simulink library "Electric_Drive_Tabled_Consumption"  (R2018b)
settings: Solver=VariableStepAuto  StartTime=0.0  StopTime=10.0  RelTol=1e-3
undefined symbols (not defined in the file): OM_PEl_M_Map, PEl_MotVector
(part 1 of 2)
settings Model: Creator=ga69qig  LastModifiedBy=ga69qig
settings SFSimCC: SimUseLocalCustomCode=off
settings RTWCC: RTWUseLocalCustomCode=off

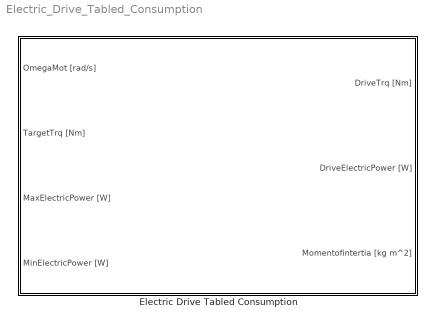
== system Electric_Drive_Tabled_Consumption ==
  Electric Drive Tabled Consumption : Subsystem  mask(SB){inertia=0.03, mass=1, OM_M_Pel_Map=[0 84.6925537915840 106.777901162710 132.451481077187 158.717445659769 189.583562564064 219.947567848300 253.359271731562 287.719734913549 325.267898465954 364.560585120281 403.200274983864 447.563591693892 492.828790386663 540.691726349864 590.166785808662 636.561358483905 684.766906055931 734.137596997731 789.985532553104 857.853179816674 908.827398035181 961.684563108046 1019.52904110769 1081.52112973929 1143.57712046773 1200.78427519799 1267.27434692366 1330.96763225908 1399.91145341150 1460.96283186014 1522.13532912128 1591.13337312260 1654.62568484686 1718.49067047593 1783.14030989899 1852.47991946389 1921.56456923299 1990.91312442103 2061.30678608583 2131.34426123832 2203.05270027821 2289.55226312012 2376.68282420177 2454.52733777355 2530.75949498243 2607.34099640618 2684.42711031811 2763.34508226637 2845.97385304829 2963.00280011347 3052.53326845787 3134.40614789669 3225.26823505504 3314.19457665049 3406.50541394017 3500.20227762135 3591.35102796290 3685.03225906601 3782.98250894227 3881.87095410315 3980.79391338854 4076.30627526000 4181.94930220964 4286.97881720375 4389.92406519024 4497.41842284860 4603.47594352982 4710.85061726193 4818.54315585332 4930.22331092001 5041.15761416958 5166.37122862945 5276.81725954101 5387.76544736434 5521.32616802780 5637.26001511646 5761.43879713315 5886.21150930422 6012.17873781274 6142.71364240950 6280.27669163038 5676.19543942961 5258.13958693589 5295.58110214479 5435.21609088646 5171.11785981694 5274.97483494523 5470.31098908416 5158.84365253269 5768.15695867421 5696.91368959506 6048.96408164810 6479.69942526134 6479.69942526134 6479.69942526134 6479.69942526134 6479.69942526134 6479.69942526134 6479.69942526134;0 84.6925537915840 106.777901162710 132.451481077187 158.717445659769 189.583562564064 219.947567848300 253.359271731562 287.719734913549 325.267898465954 364.560585120281 403.200274983864 447.563591693892 492.828790386663 540.691726349864 590.166785808662 636.561358483905 684.766906055931 734.137596997731 789.985532553104 857.853179816674 908.827398035181 961.684563108046 1019.52904110769 1081.52112973929 1143.57712046773 1200.78427519799 1267.27434692366 1330.96763225908 1399.91145341150 1460.96283186014 1522.13532912128 1591.13337312260 1654.62568484686 1718.49067047593 1783.14030989899 1852.47991946389 1921.56456923299 1990.91312442103 2061.30678608583 2131.34426123832 2203.05270027821 2289.55226312012 2376.68282420177 2454.52733777355 2530.75949498243 2607.34099640618 2684.42711031811 2763.34508226637 2845.97385304829 2963.00280011347 3052.53326845787 3134.40614789669 3225.26823505504 3314.19457665049 3406.50541394017 3500.20227762135 3591.35102796290 3685.03225906601 3782.98250894227 3881.87095410315 3980.79391338854 4076.30627526000 4181.94930220964 4286.97881720375 4389.92406519024 4497.41842284860 4603.47594352982 4710.85061726193 4818.54315585332 4930.22331092001 5041.15761416958 5166.37122862945 5276.81725954101 5387.76544736434 5521.32616802780 5637.26001511646 5761.43879713315 5886.21150930422 6012.17873781274 6142.71364240950 6280.27669163038 5676.19543942961 5258.13958693589 5295.58110214479 5435.21609088646 5171.11785981694 5274.97483494523 5470.31098908416 5158.84365253269 5768.15695867421 5696.91368959506 6048.96408164810 6479.69942526134 6479.69942526134 6479.69942526134 6479.69942526134 6479.69942526134 6479.69942526134 6479.69942526134;0 84.6925537915840 106.777901162710 132.451481077187 158.717445659769 189.583562564064 219.947567848300 253.359271731562 287.719734913549 325.267898465954 364.560585120281 403.200274983864 447.563591693892 492.828790386663 540.691726349864 590.166785808662 636.561358483905 684.766906055931 734.137596997731 789.985532553104 857.853179816674 908.827398035181 961.684563108046 1019.52904110769 1081.52112973929 1143.57712046773 1200.78427519799 1267.27434692366 1330.96763225908 1399.91145341150 1460.96283186014 1522.13532912128 1591.13337312260 1654.62568484686 1718.49067047593 1783.14030989899 1852.47991946389 ...(+366716 chars)], M_MotVector=[0 1.36363636363636 2.72727272727273 4.09090909090909 5.45454545454545 6.81818181818182 8.18181818181818 9.54545454545455 10.9090909090909 12.2727272727273 13.6363636363636 15.0000000000000 16.3636363636364 17.7272727272727 19.0909090909091 20.4545454545455 21.8181818181818 23.1818181818182 24.5454545454545 25.9090909090909 27.2727272727273 28.6363636363636 30.0000000000000 31.3636363636364 32.7272727272727 34.0909090909091 35.4545454545455 36.8181818181818 38.1818181818182 39.5454545454545 40.9090909090909 42.2727272727273 43.6363636363636 45 46.3636363636364 47.7272727272727 49.0909090909091 50.4545454545455 51.8181818181818 53.1818181818182 54.5454545454545 55.9090909090909 57.2727272727273 58.6363636363636 60.0000000000000 61.3636363636364 62.7272727272727 64.0909090909091 65.4545454545455 66.8181818181818 68.1818181818182 69.5454545454546 70.9090909090909 72.2727272727273 73.6363636363636 75 76.3636363636364 77.7272727272727 79.0909090909091 80.4545454545455 81.8181818181818 83.1818181818182 84.5454545454546 85.9090909090909 87.2727272727273 88.6363636363636 90 91.3636363636364 92.7272727272727 94.0909090909091 95.4545454545455 96.8181818181818 98.1818181818182 99.5454545454546 100.909090909091 102.272727272727 103.636363636364 105 106.363636363636 107.727272727273 109.090909090909 110.454545454545 111.818181818182 113.181818181818 114.545454545455 115.909090909091 117.272727272727 118.636363636364 120 121.363636363636 122.727272727273 124.090909090909 125.454545454545 126.818181818182 128.181818181818 129.545454545455 130.909090909091 132.272727272727 133.636363636364 135], OM_MotVector=[0 3.13202920563366 6.26405841126732 9.39608761690098 12.5281168225346 15.6601460281683 18.7921752338020 21.9242044394356 25.0562336450693 28.1882628507029 31.3202920563366 34.4523212619703 37.5843504676039 40.7163796732376 43.8484088788712 46.9804380845049 50.1124672901386 53.2444964957722 56.3765257014059 59.5085549070395 62.6405841126732 65.7726133183069 68.9046425239405 72.0366717295742 75.1687009352078 78.3007301408415 81.4327593464752 84.5647885521088 87.6968177577425 90.8288469633761 93.9608761690098 97.0929053746435 100.224934580277 103.356963785911 106.488992991544 109.621022197178 112.753051402812 115.885080608445 119.017109814079 122.149139019713 125.281168225346 128.413197430980 131.545226636614 134.677255842247 137.809285047881 140.941314253515 144.073343459148 147.205372664782 150.337401870416 153.469431076049 156.601460281683 159.733489487317 162.865518692950 165.997547898584 169.129577104218 172.261606309851 175.393635515485 178.525664721119 181.657693926752 184.789723132386 187.921752338020 191.053781543653 194.185810749287 197.317839954921 200.449869160554 203.581898366188 206.713927571822 209.845956777455 212.977985983089 216.110015188723 219.242044394356 222.374073599990 225.506102805624 228.638132011257 231.770161216891 234.902190422524 238.034219628158 241.166248833792 244.298278039425 247.430307245059 250.562336450693 253.694365656326 256.826394861960 259.958424067594 263.090453273227 266.222482478861 269.354511684495 272.486540890128 275.618570095762 278.750599301396 281.882628507029 285.014657712663 288.146686918297 291.278716123930 294.410745329564 297.542774535198 300.674803740831 303.806832946465 306.938862152099 310.070891357732 313.202920563366 316.334949769000 319.466978974633 322.599008180267 325.731037385901 328.863066591534 331.995095797168 335.127125002802 338.259154208435 341.391183414069 344.523212619703 347.655241825336 350.787271030970 353.919300236604 357.051329442237 360.183358647871 363.315387853505 366.447417059138 369.579446264772 372.711475470406 375.843504676039 378.975533881673 382.107563087307 385.239592292940 388.371621498574 391.503650704208 394.635679909841 397.767709115475 400.899738321108 404.031767526742 407.163796732376 410.295825938009 413.427855143643 416.559884349277 419.691913554910 422.823942760544 425.955971966178 429.088001171811 432.220030377445 435.352059583079 438.484088788712 441.616117994346 444.748147199980 447.880176405613 451.012205611247 454.144234816881 457.276264022514 460.408293228148 463.540322433782 466.672351639415 469.804380845049 472.936410050683 476.068439256316 479.200468461950 482.332497667584 485.464526873217 488.596556078851 491.728585284485 494.860614490118 497.992643695752 501.124672901386 504.256702107019 507.388731312653 510.520760518287 513.652789723920 516.784818929554 519.916848135188 523.048877340821 526.180906546455 529.312935752089 532.444964957722 535.576994163356 538.709023368990 541.841052574623 544.973081780257 548.105110985890 551.237140191524 554.369169397158 557.501198602791 560.633227808425 563.765257014059 566.897286219692 570.029315425326 573.161344630960 576.293373836593 579.425403042227 582.557432247861 585.689461453494 588.821490659128 591.953519864762 595.085549070395 598.217578276029 601.349607481663 604.481636687296 607.613665892930 610.745695098564 613.877724304197 617.009753509831 620.141782715465 623.273811921098 626.405841126732 629.537870332366 632.669899537999 635.801928743633 638.933957949267 642.065987154900 645.198016360534 648.330045566168 651.462074771801 654.594103977435 657.726133183069 660.858162388702 663.990191594336 667.122220799970 670.254250005603 673.386279211237 676.518308416871 679.650337622504 682.782366828138 685.914396033772], M_Full_Load=[128 128 128 127 127 126 126 126 126 124 119 114 109 103 100 94 89 85 79 75 70 68 67 65 63 62 60 58 59 60 62 63 63 62 61 60 58 57 55 53 51 50 48 46 45 43 42 40 39 38 36 35 34 32 31 30 29 28 26 25 24], OM_Full_Load=[0 11.4144533080429 22.8289066160858 34.2433599241288 45.6578132321717 57.1769862953342 68.5914396033771 80.0058929114201 91.4203462194630 102.834799527506 114.249252835549 125.663706143592 137.078159451635 148.492612759678 160.011785822840 171.426239130883 182.840692438926 194.255145746969 205.669599055012 217.084052363055 228.498505671098 239.912958979141 251.327412287183 262.846585350346 274.261038658389 285.675491966432 297.089945274475 308.504398582518 319.918851890561 331.333305198604 342.747758506646 354.162211814689 365.681384877852 377.095838185895 388.510291493938 399.924744801981 411.339198110024 422.753651418066 434.168104726109 445.582558034152 456.997011342195 468.516184405358 479.930637713401 491.345091021444 502.759544329487 514.173997637529 525.588450945572 537.002904253615 548.417357561658 559.831810869701 571.350983932864 582.765437240907 594.179890548950 605.594343856992 617.008797165035 628.423250473078 639.837703781121 651.252157089164 662.666610397207 674.185783460370 685.600236768413], M_Min_Load=[0 0 0 0 0 0 0 0 0 0 0 0 0 0 0 0 0 0 0 0 0 0 0 0 0 0 0 0 0 0 0 0 0 0 0 0 0 0 0 0 0 0 0 0 0 0 0 0 0 0 0 0 0 0 0 0 0 0 0 0 0], OM_Min_Load=[0 11.4144533080429 22.8289066160858 34.2433599241288 45.6578132321717 57.1769862953342 68.5914396033771 80.0058929114201 91.4203462194630 102.834799527506 114.249252835549 125.663706143592 137.078159451635 148.492612759678 160.011785822840 171.426239130883 182.840692438926 194.255145746969 205.669599055012 217.084052363055 228.498505671098 239.912958979141 251.327412287183 262.846585350346 274.261038658389 285.675491966432 297.089945274475 308.504398582518 319.918851890561 331.333305198604 342.747758506646 354.162211814689 365.681384877852 377.095838185895 388.510291493938 399.924744801981 411.339198110024 422.753651418066 434.168104726109 445.582558034152 456.997011342195 468.516184405358 479.930637713401 491.345091021444 502.759544329487 514.173997637529 525.588450945572 537.002904253615 548.417357561658 559.831810869701 571.350983932864 582.765437240907 594.179890548950 605.594343856992 617.008797165035 628.423250473078 639.837703781121 651.252157089164 662.666610397207 674.185783460370 685.600236768413], LocalSampleTime=-1}
      mask prompts: inertia "Moment of Inertia E-Motor [kg*m^2]"; mass "Mass E-Motor [kg"; OM_M_Pel_Map "Tabled Electric Power [NxM]"; M_MotVector "Reference Torque Vector [1xM]"; OM_MotVector "Reference Omega Vector [1xN]"; M_Full_Load "Torque Vector for Full Load Line [1xL]"; OM_Full_Load "Reference Omega Vector for Full Load Line [1xL]"; M_Min_Load "Torque Vector for Min Load Line [1xK]"; OM_Min_Load "Reference Omega Vector for Min Load Line [1xK]"; LocalSampleTime "Local System Sample-Time [s]"
      mask help:
      | <Author> Benedikt Danquah based on Lorenz Horlbeck [1] and Philip Wacker [2]</Author>
      | <Date> 01/2019 </Date>
      |
      | <Description>
      | Calculates the target drive torque. The avaiable max./min. electric power of the battery limits the electric system. The mechanical system is limited by the max./min. torque curve. Due to the limits the final drive torque and the drive electric power (via 2D-Lookup table) is calculated. The moment of inertia is given as a constant signal.
      | </Description>
      mask init:
      | GlobalSampleTime = CalcGlobalSampleTime(LocalSampleTime);
      | 
      | [OM_PEl_M_Map,OM_MotVector, PEl_MotVector]= init_Electric_Drive_Tabled_Consumption (OM_M_Pel_Map,M_MotVector,OM_MotVector,M_Full_Load,OM_Full_Load,M_Min_Load,OM_Min_Load);
      | 
      | %figure
      | %hold on
      | %surfc(OM_MotVector,M_MotVector,OM_M_Pel_Map')
      | %for i=1:1000
      |  %   plot3(OM_Full_Load,M_Full_Load,ones(1,61)*i*30,'color','red', 'linewidth',6)
      | %end
      | %hold off
      | 
      | 
      | %figure
      | %surfc(OM_MotVector,PEl_Vector,OM_PEl_M_Map')
      mask Help:
      | <Parameters>
      | Moment of Inertia E-Motor [kg*m^2]
      | Mass E-Motor [kg]
      | Tabled Electric Power [NxM]
      | Reference Torque Vector [1xM]
      | Reference Omega Vector [1xN]
      | Torque Vector for Full Load Line [1xL]
      | Reference Omega Vector for Full Load Line [1xL]
      | Torque Vector for Min Load Line [1xK]
      | Reference Omega Vector for Min Load Line [1xK]
      | </Parameters>
      | 
      | with M,N,P = ∈ {ℕ}
      | 
      | <Inputs>
      | OmegaMot [rad/s]
      | TargetTrq [Nm]
      | MaxElectricPower [W]
      | 	<sign orientation> [+] discharge </sign orientation>
      | MinElectricPower  [W]
      | 	<sign orientation> [-] charge </sign orientation>
      | </Inputs>
      | 
      | <Outputs>
      | DriveTrq [Nm]
      | DriveElectricPower [W]
      | 	<sign orientation> [+] discharge </sign orientation>
      | Momentofinertia [kg*m^2]
      | </Outputs>
      | <Sources>
      | [1] L. Horlbeck, “Auslegung elektrischer Maschinen für automobile Antriebsstränge unter Berücksichtigung des Überlastpotentials,” Dissertation, Institute of Automotive Technology, Technical University Munich, Munich, 2018.
      | [2] P. Wacker, J. Adermann, B. Danquah, and M. Lienkamp, “Efficiency determination of active battery switching technology on roller dynamometer,” in Twelfth International Conference on Ecological Vehicles and Renewable Energies, Monaco, 2017, pp. 1–7.
      | </Sources>
      mask TypeOptions LocalSampleTime: OmegaMot [rad//s]/SampleTime | TargetTrq [Nm]/SampleTime | MaxElectricPower [W]/SampleTime | MinElectricPower [W]/SampleTime
      mask DialogControl Container3 Prompt: Documentation
      mask DialogControl Control4 Prompt: %<MaskHelp>
      mask DialogControl show_plot Prompt: Plot Consumption Map
      mask DialogControl show_plot Callback: PlotMaps(gcb);
      mask DialogControl Container7 Prompt: Sample Time
      mask Display:
      | [picturexpos,pictureypos,picturewidth,pictureheight] = ...
      |     CalcBlockPicturePosition(gcb,1,0.01,0.1,100,100); % calculating picture position depending on Block size and minimum margin size
      | image('Electric_Drive_Tabled_Consumption.svg',[picturexpos pictureypos picturewidth pictureheight]) % plot picture to block
